simulink model "Chopper_with_DCSource_with_ElectricalComponents"  (R2016a)
settings: Solver=VariableStepAuto  StartTime=0.0  StopTime=0.9  RelTol=1e-3
libraries: fl_lib x18, nesl_utility x10, elec_lib x6, pe_lib x4, powerlib_meascontrol x1
settings Model: Creator=kkfrk  LastModifiedBy=kkfrk

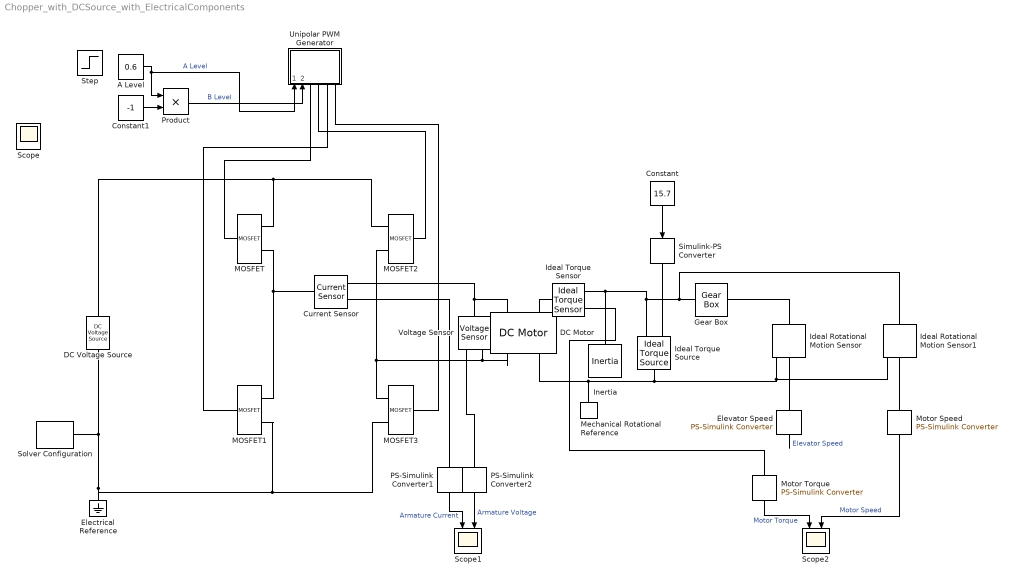
== system Chopper_with_DCSource_with_ElectricalComponents ==
  A Level : Constant  Value=0.6
  Constant : Constant  Value=15.7
  Constant1 : Constant  Value=-1
  Current Sensor : fl_lib/Electrical/Electrical Sensors/Current Sensor
  DC Motor : elec_lib/Actuators & Drivers/Rotational Actuators/DC Motor  parameterization=1  Ra=3.68 Ohm  La=32e-3 H  emf_or_torque=1  Kv=1.66 V/(rad/s)  Ki=6.876e-4 N*m/A  T_stall=2.4e-4 N*m  w_max=1.91e+4 rpm  w_rated=1.5e+4 rpm  P_rated=0.08 W  V_rated=1.5 V  J=0.05 kg*m^2  lam_param=1  lam=0 N*m/(rad/s)  i_noload=0 A  V_i_noload=1.5 V  speed0=0 rpm  alpha=0.00393 1/K  Tmeas=25 degC  thermal_mass=100 J/K  initial_temperature=25 degC
  DC Voltage Source : elec_lib/Additional Components/SPICE-Compatible Components/Sources/DC Voltage Source  DC=537.8 V
  Electrical Reference : fl_lib/Electrical/Electrical Elements/Electrical Reference
  Elevator Speed : nesl_utility/PS-Simulink Converter  PhysicalDomain=network_engine_domain  SubClassName=ps_output  LeftPortType=input  RightPortType=output  PseudoPeriodic=off  Frequencies=[]  Unit=1  AffineConversion=off
  Gear Box : fl_lib/Mechanical/Mechanisms/Gear Box  ratio=12.5  t_in_specify=off  t_in_priority=None  t_in=0 N*m  t_out_specify=off  t_out_priority=None  t_out=0 N*m
  Ideal Rotational Motion Sensor : fl_lib/Mechanical/Mechanical Sensors/Ideal Rotational Motion Sensor  offset=0 rad
  Ideal Rotational Motion Sensor1 : fl_lib/Mechanical/Mechanical Sensors/Ideal Rotational Motion Sensor  offset=0 rad
  Ideal Torque Sensor : fl_lib/Mechanical/Mechanical Sensors/Ideal Torque Sensor
  Ideal Torque Source : fl_lib/Mechanical/Mechanical Sources/Ideal Torque Source
  Inertia : fl_lib/Mechanical/Rotational Elements/Inertia  inertia=0.0512 kg*m^2  w_specify=off  w_priority=High  w=0 rad/s  t_specify=off  t_priority=None  t=0 N*m
  MOSFET{,1..3} (4 alike) : pe_lib/Semiconductors/Fundamental Components/MOSFET  Rds=0.001 Ohm  Goff=1e-6 1/Ohm  Vth=1.1 V  diode_param=2  diode_Vf=0.8 V  diode_Ron=0.001 Ohm  diode_Goff=1e-5 1/Ohm  diode_C=5e-8 F  diode_iRM=-235 A  diode_iF=300 A  diode_idot=-50 A/us  diode_trr_param=1  diode_trr_factor=3  diode_trr=15 us  diode_Qrr=1.5e+3 s*uA
  Mechanical Rotational Reference : fl_lib/Mechanical/Rotational Elements/Mechanical Rotational Reference
  Motor Speed : nesl_utility/PS-Simulink Converter  PhysicalDomain=network_engine_domain  SubClassName=ps_output  LeftPortType=input  RightPortType=output  PseudoPeriodic=off  Frequencies=[]  Unit=1  AffineConversion=off
  Motor Torque : nesl_utility/PS-Simulink Converter  PhysicalDomain=network_engine_domain  SubClassName=ps_output  LeftPortType=input  RightPortType=output  PseudoPeriodic=off  Frequencies=[]  Unit=1  AffineConversion=off
  PS-Simulink Converter1 : nesl_utility/PS-Simulink Converter  PhysicalDomain=network_engine_domain  SubClassName=ps_output  LeftPortType=input  RightPortType=output  PseudoPeriodic=off  Frequencies=[]  Unit=1  AffineConversion=off
  PS-Simulink Converter2 : nesl_utility/PS-Simulink Converter  PhysicalDomain=network_engine_domain  SubClassName=ps_output  LeftPortType=input  RightPortType=output  PseudoPeriodic=off  Frequencies=[]  Unit=1  AffineConversion=off
  Product : Product
  Scope1 : Scope  NumInputPorts=2
  Scope2 : Scope  NumInputPorts=2
  Simulink-PS Converter : nesl_utility/Simulink-PS Converter  PhysicalDomain=network_engine_domain  SubClassName=ps_input  LeftPortType=input  RightPortType=output  PseudoPeriodic=off  Frequencies=[]  NoiseDistribution=none  NoiseParameters=[]  Unit=1  AffineConversion=off  InputFiltering=off  SimscapeFilterOrder=1  InputFilterTimeConstant=0.001  UdotUserProvided=1
  Solver Configuration : nesl_utility/Solver Configuration  PhysicalDomain=network_engine_domain  SubClassName=solver  LeftPortType=input  RightPortType=generic  Accelerate=off  Tones=[]  Harmonics=[]  SimulateNoise=off  Profile=off  UseLocalSampling=off  EnableSwitchedLinearOptims=on  FrequencyDomain=off  UseCCode=off  RelTol=0.001  AbsTol=1e-06  MinStep=1e-09  ToWorkspace=off  RevertToSquareIcSolve=off  NumHomotopyIterations=100  PhasorMode=off  PhasorModeNumHarmonics=1  OverrideAbsTol=off  DoDC=off  ResidualTolerance=1e-09  UseLocalSolver=on  LocalSolverChoice=NE_BACKWARD_EULER_ADVANCER  LocalSolverSampleTime=0.000001  DoFixedCost=on  MaxNonlinIter=3  MaxModeIter=2  LinearAlgebra=Sparse  DelaysMemoryBudget=10*4096  AutomaticFiltering=on  FilteringTimeConstant=0.001
  Step : Step  Before=0.6  After=-0.6  SampleTime=0
  Unipolar PWM Generator : Subsystem
  Voltage Sensor : fl_lib/Electrical/Electrical Sensors/Voltage Sensor
  Scope : Scope
  wires:
  Constant/1 -> Simulink-PS Converter/1
  Product/1 -> Unipolar PWM Generator/2(In2)  "B Level"
  PS-Simulink Converter2/1 -> Scope1/2  "Armature Voltage"
  PS-Simulink Converter1/1 -> Scope1/1  "Armature Current"
  Elevator Speed/1 -> ?  "Elevator Speed"
  Motor Speed/1 -> Scope2/2  "Motor Speed"
  Motor Torque/1 -> Scope2/1  "Motor Torque"
  Constant1/1 -> Product/2
  A Level/1 -> Unipolar PWM Generator/1(In1), Product/1  "A Level"
  connections:
  MOSFET/RConn1 -- MOSFET2/RConn1 -- DC Voltage Source/LConn1
  MOSFET1/RConn1 -- Current Sensor/LConn1 -- MOSFET/RConn2
  MOSFET3/RConn1 -- Voltage Sensor/RConn2 -- DC Motor/RConn1 -- MOSFET2/RConn2
  DC Voltage Source/RConn1 -- Solver Configuration/RConn1 -- MOSFET1/RConn2 -- MOSFET3/RConn2 -- Electrical Reference/LConn1
  Ideal Torque Sensor/LConn1 -- DC Motor/LConn2
  Ideal Rotational Motion Sensor/LConn1 -- Gear Box/RConn1
  DC Motor/RConn2 -- Ideal Rotational Motion Sensor1/RConn1 -- Ideal Rotational Motion Sensor/RConn1 -- Ideal Torque Source/LConn1 -- Mechanical Rotational Reference/LConn1
  Simulink-PS Converter/RConn1 -- Ideal Torque Source/RConn1
  Elevator Speed/LConn1 -- Ideal Rotational Motion Sensor/RConn2
  Unipolar PWM Generator/LConn1 -- MOSFET/LConn1
  Unipolar PWM Generator/LConn2 -- MOSFET2/LConn1
  Unipolar PWM Generator/LConn3 -- MOSFET1/LConn1
  Unipolar PWM Generator/LConn4 -- MOSFET3/LConn1
  DC Motor/LConn1 -- Voltage Sensor/LConn1 -- Current Sensor/RConn2
  PS-Simulink Converter1/LConn1 -- Current Sensor/RConn1
  PS-Simulink Converter2/LConn1 -- Voltage Sensor/RConn1
  Ideal Rotational Motion Sensor1/RConn2 -- Motor Speed/LConn1
  Ideal Rotational Motion Sensor1/LConn1 -- Inertia/LConn1 -- Ideal Torque Sensor/RConn1 -- Ideal Torque Source/RConn2 -- Gear Box/LConn1
  Ideal Torque Sensor/RConn2 -- Motor Torque/LConn1

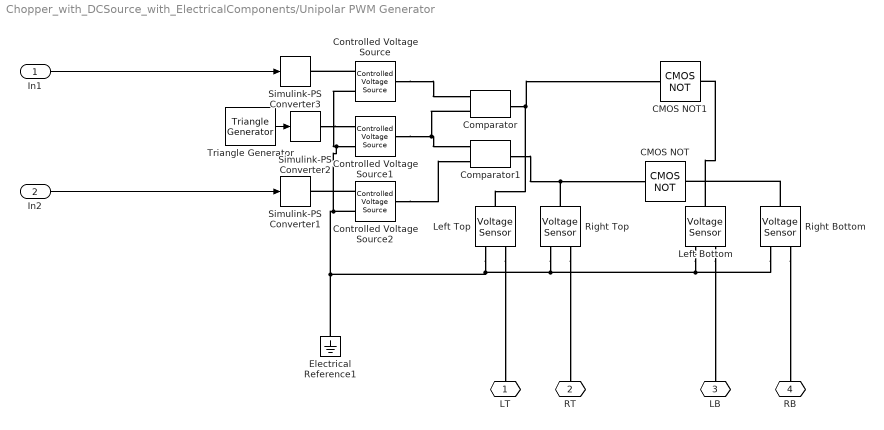
== system Chopper_with_DCSource_with_ElectricalComponents/Unipolar PWM Generator ==
  In1 : Inport
  In2 : Inport  Port=2
  CMOS NOT : elec_lib/Integrated Circuits/Logic/CMOS NOT  V_IL=1 V  V_IH=10 V  C_IN=5 pF  output_type=1  V_OL=0 V  V_OH=10 V  V_CC=5 V  V_meas=5 V  R_OUT=25 Ohm  R_OH=[ 25 250 ] Ohm  I_OH=63 mA  R_OL=[ 30 800 ] Ohm  I_OL=-45 mA  Delay=25 ns  Ron=5 Ohm  Vf=0.6 V  output_state=1
  CMOS NOT1 : elec_lib/Integrated Circuits/Logic/CMOS NOT  V_IL=1 V  V_IH=10 V  C_IN=5 pF  output_type=1  V_OL=0 V  V_OH=10 V  V_CC=5 V  V_meas=5 V  R_OUT=25 Ohm  R_OH=[ 25 250 ] Ohm  I_OH=63 mA  R_OL=[ 30 800 ] Ohm  I_OL=-45 mA  Delay=25 ns  Ron=5 Ohm  Vf=0.6 V  output_state=1
  Comparator : elec_lib/Integrated Circuits/Comparator  V_OS=1 mV  V_OL=1 V  V_OH=10 V  C_IN=0 pF  R_OUT=50 Ohm  Delay=0 s
  Comparator1 : elec_lib/Integrated Circuits/Comparator  V_OS=1 mV  V_OL=1 V  V_OH=10 V  C_IN=0 pF  R_OUT=50 Ohm  Delay=0 s
  Controlled Voltage Source : fl_lib/Electrical/Electrical Sources/Controlled Voltage Source
  Controlled Voltage Source1 : fl_lib/Electrical/Electrical Sources/Controlled Voltage Source
  Controlled Voltage Source2 : fl_lib/Electrical/Electrical Sources/Controlled Voltage Source
  Electrical Reference1 : fl_lib/Electrical/Electrical Elements/Electrical Reference
  Left Bottom : fl_lib/Electrical/Electrical Sensors/Voltage Sensor
  Left Top : fl_lib/Electrical/Electrical Sensors/Voltage Sensor
  Right Bottom : fl_lib/Electrical/Electrical Sensors/Voltage Sensor
  Right Top : fl_lib/Electrical/Electrical Sensors/Voltage Sensor
  Simulink-PS Converter1 : nesl_utility/Simulink-PS Converter  PhysicalDomain=network_engine_domain  SubClassName=ps_input  LeftPortType=input  RightPortType=output  PseudoPeriodic=off  Frequencies=[]  NoiseDistribution=none  NoiseParameters=[]  Unit=1  AffineConversion=off  InputFiltering=off  SimscapeFilterOrder=1  InputFilterTimeConstant=0.001  UdotUserProvided=1
  Simulink-PS Converter2 : nesl_utility/Simulink-PS Converter  PhysicalDomain=network_engine_domain  SubClassName=ps_input  LeftPortType=input  RightPortType=output  PseudoPeriodic=off  Frequencies=[]  NoiseDistribution=none  NoiseParameters=[]  Unit=1  AffineConversion=off  InputFiltering=off  SimscapeFilterOrder=1  InputFilterTimeConstant=0.001  UdotUserProvided=1
  Simulink-PS Converter3 : nesl_utility/Simulink-PS Converter  PhysicalDomain=network_engine_domain  SubClassName=ps_input  LeftPortType=input  RightPortType=output  PseudoPeriodic=off  Frequencies=[]  NoiseDistribution=none  NoiseParameters=[]  Unit=1  AffineConversion=off  InputFiltering=off  SimscapeFilterOrder=1  InputFilterTimeConstant=0.001  UdotUserProvided=1
  Triangle Generator : powerlib_meascontrol/Pulse & Signal Generators/Triangle Generator  Freq=15e3  Phase=90  Ts=0
  LT : PMIOPort  Port=1  Side=Left
  RT : PMIOPort  Port=2  Side=Left
  LB : PMIOPort  Port=3  Side=Left
  RB : PMIOPort  Port=4  Side=Left
  wires:
  In2/1 -> Simulink-PS Converter1/1
  In1/1 -> Simulink-PS Converter3/1
  Triangle Generator/1 -> Simulink-PS Converter2/1
  connections:
  Controlled Voltage Source/RConn2 -- Right Bottom/RConn2 -- Left Bottom/RConn2 -- Right Top/RConn2 -- Left Top/RConn2 -- Electrical Reference1/LConn1 -- Controlled Voltage Source2/RConn2 -- Controlled Voltage Source1/RConn2
  Left Bottom/LConn1 -- CMOS NOT1/RConn1
  Controlled Voltage Source2/LConn1 -- Comparator1/LConn1
  Left Bottom/RConn1 -- LB/RConn1
  Comparator/RConn1 -- Left Top/LConn1 -- CMOS NOT1/LConn1
  Controlled Voltage Source/RConn1 -- Simulink-PS Converter3/RConn1
  Left Top/RConn1 -- LT/RConn1
  Right Top/RConn1 -- RT/RConn1
  Right Bottom/RConn1 -- RB/RConn1
  Controlled Voltage Source/LConn1 -- Comparator/LConn1
  Controlled Voltage Source2/RConn1 -- Simulink-PS Converter1/RConn1
  Controlled Voltage Source1/LConn1 -- Comparator/LConn2 -- Comparator1/LConn2
  Simulink-PS Converter2/RConn1 -- Controlled Voltage Source1/RConn1
  Comparator1/RConn1 -- Right Top/LConn1 -- CMOS NOT/LConn1
  Right Bottom/LConn1 -- CMOS NOT/RConn1
